simulink model "sh_harness"  (R2021b)
settings: Solver=VariableStepAuto  StartTime=0.0  StopTime=t_stop  FixedStep=1e-3  RelTol=1e-3
values from neighbouring files (symbols this model uses):
  Gr = 2.56e-6    (= 2.56e-06)    [skyhook.m]
  test_vehicle = 0    [skyhook.m]
  test_wheel = 1    [skyhook.m]
  user_enable = 1    [skyhook.m]
  v_car = 30/3.6    (= 8.33333333333)    [skyhook.m]
libraries: simulink x1
settings Model: Creator=Luca  LastModifiedBy=Luca
settings DataIOCC: ReturnWorkspaceOutputs=off

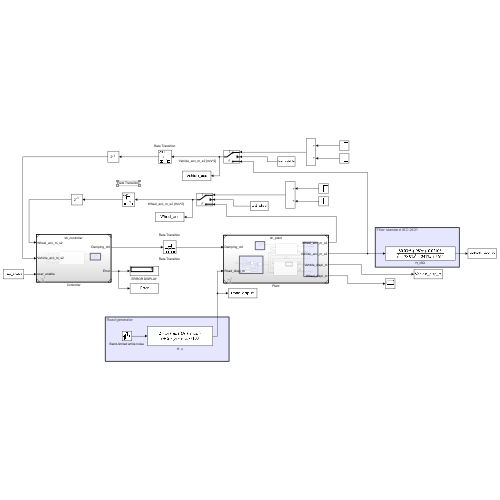
[thumbnail: Simulink's stored preview of the top-level diagram]
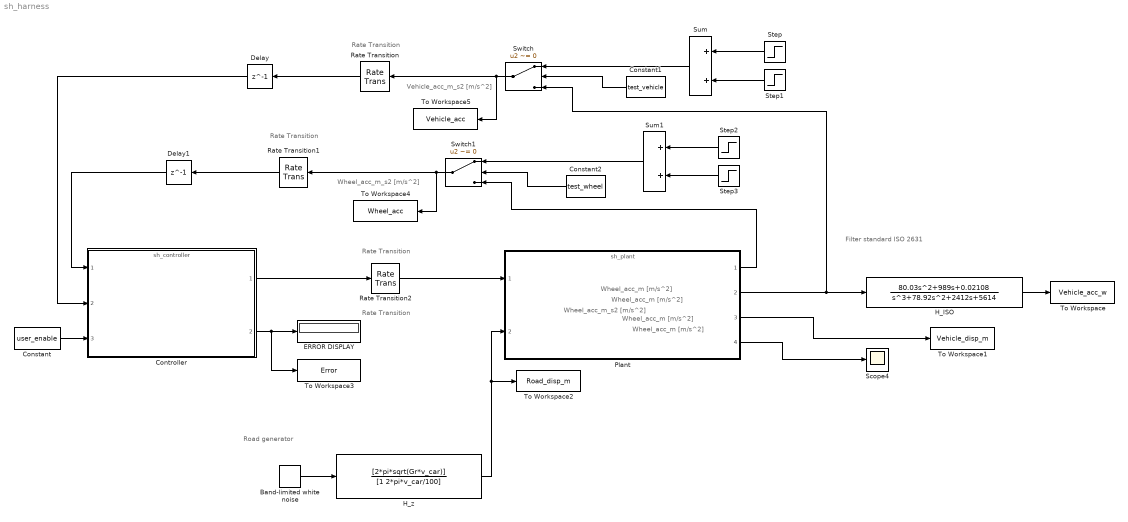
== system sh_harness ==
  note: Wheel_acc_m_s2 [m/s^2]
  note: Wheel_acc_m_s2 [m/s^2]
  note: Wheel_acc_m [m/s^2]
  note: Wheel_acc_m [m/s^2]
  note: Wheel_acc_m [m/s^2]
  note: Wheel_acc_m [m/s^2]
  note: Vehicle_acc_m_s2 [m/s^2]
  note: Rate Transition
  note: Rate Transition
  note: Rate Transition
  note: Road generator
  note: Filter standard ISO 2631
  note: Rate Transition
  Band-limited white noise : simulink/Sources/Band-Limited White Noise  Cov=[0.5]  Ts=1e-3  seed=[23347]
  Constant : Constant  Value=user_enable  OutDataTypeStr=boolean
  Constant1 : Constant  Value=test_vehicle  OutDataTypeStr=boolean
  Constant2 : Constant  Value=test_wheel  OutDataTypeStr=boolean
  Controller : ModelReference  ModelNameDialog=sh_controller.slx  SimulationMode=Normal  ModelReferenceVersion=1.27
  Delay : Delay  DelayLength=1
  Delay1 : Delay  DelayLength=1
  ERROR DISPLAY : Display
  H_ISO : TransferFcn  Numerator=[80.03 989 0.02108]  Denominator=[1 78.92 2412 5614]
  H_z : TransferFcn  Numerator=[2*pi*sqrt(Gr*v_car)]  Denominator=[1 2*pi*v_car/100]
  Plant : ModelReference  ModelNameDialog=sh_plant.slx  SimulationMode=Normal  ModelReferenceVersion=1.60
  Rate Transition : RateTransition
  Rate Transition1 : RateTransition
  Rate Transition2 : RateTransition
  Scope4 : Scope
  Step : Step  Time=10e-3  SampleTime=0
  Step1 : Step  Time=31e-3  After=-1  SampleTime=0
  Step2 : Step  Time=10e-3  SampleTime=0
  Step3 : Step  Time=31e-3  After=-1  SampleTime=0
  Sum : Sum
  Sum1 : Sum
  Switch : Switch  Criteria=u2 ~= 0
  Switch1 : Switch  Criteria=u2 ~= 0
  To Workspace : ToWorkspace  VariableName=Vehicle_acc_w  SaveFormat=Timeseries  SampleTime=-1
  To Workspace1 : ToWorkspace  VariableName=Vehicle_disp_m  SaveFormat=Timeseries  SampleTime=-1
  To Workspace2 : ToWorkspace  VariableName=Road_disp_m  SaveFormat=Timeseries  SampleTime=-1
  To Workspace3 : ToWorkspace  VariableName=Error  SaveFormat=Timeseries  SampleTime=-1
  To Workspace4 : ToWorkspace  VariableName=Wheel_acc  SaveFormat=Timeseries  SampleTime=-1
  To Workspace5 : ToWorkspace  VariableName=Vehicle_acc  SaveFormat=Timeseries  SampleTime=-1
  wires:
  Controller/2 -> To Workspace3/1, ERROR DISPLAY/1
  Plant/3 -> To Workspace1/1
  Plant/4 -> Scope4/1
  Plant/2 -> Switch/3, H_ISO/1
  Band-limited white noise/1 -> H_z/1
  H_z/1 -> To Workspace2/1, Plant/2
  H_ISO/1 -> To Workspace/1
  Controller/1 -> Rate Transition2/1
  Rate Transition/1 -> Delay/1
  Rate Transition1/1 -> Delay1/1
  Rate Transition2/1 -> Plant/1
  Delay/1 -> Controller/2
  Delay1/1 -> Controller/1
  Constant/1 -> Controller/3
  Step1/1 -> Sum/2
  Step/1 -> Sum/1
  Switch/1 -> To Workspace5/1, Rate Transition/1
  Constant1/1 -> Switch/2
  Sum/1 -> Switch/1
  Sum1/1 -> Switch1/1
  Switch1/1 -> To Workspace4/1, Rate Transition1/1
  Step3/1 -> Sum1/2
  Constant2/1 -> Switch1/2
  Step2/1 -> Sum1/1
  Plant/1 -> Switch1/3
